simulink model "p2Sim"  (R2019a)
settings: Solver=ode1  StartTime=0.0  StopTime=s.TFinal  FixedStep=s.Tstep  RelTol=1e-3
undefined symbols (not defined in the file): d, kdc, Ki, Kp, mytfpl, s, tau, tau2
settings Model: Creator=vtaware  LastModifiedBy=vtaware

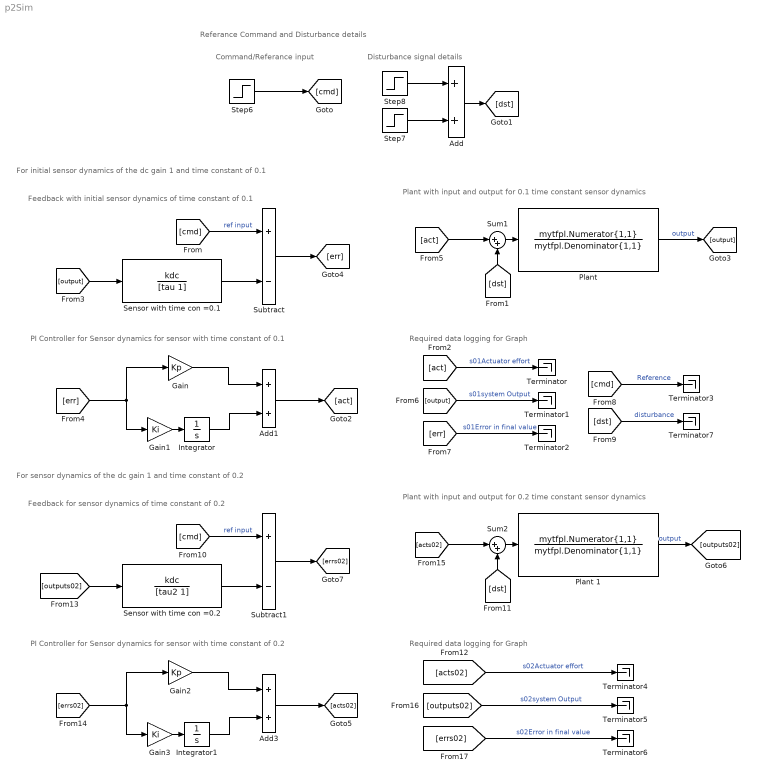
== system p2Sim ==
  note: Referance Command and Disturbance details
  note: Required data logging for Graph
  note: For initial sensor dynamics of the dc gain 1 and time constant of 0.1
  note: Plant with input and output for 0.1 time constant sensor dynamics
  note: Feedback with initial sensor dynamics of time constant of 0.1
  note: PI Controller for Sensor dynamics for sensor with time constant of 0.1
  note: Disturbance signal details
  note: Command/Referance input
  note: Required data logging for Graph
  note: For sensor dynamics of the dc gain 1 and time constant of 0.2
  note: Plant with input and output for 0.2 time constant sensor dynamics
  note: Feedback for sensor dynamics of time constant of 0.2
  note: PI Controller for Sensor dynamics for sensor with time constant of 0.2
  Add : Sum
  Add1 : Sum
  Add3 : Sum
  Gain : Gain  Gain=Kp
  Gain1 : Gain  Gain=Ki
  Gain2 : Gain  Gain=Kp
  Gain3 : Gain  Gain=Ki
  Integrator : Integrator
  Integrator1 : Integrator
  "Plant " : TransferFcn  Numerator=mytfpl.Numerator{1,1}  Denominator=mytfpl.Denominator{1,1}
  Plant 1 : TransferFcn  Numerator=mytfpl.Numerator{1,1}  Denominator=mytfpl.Denominator{1,1}
  Sensor with time con =0.1 : TransferFcn  Numerator=kdc  Denominator=[tau 1]
  Sensor with time con =0.2 : TransferFcn  Numerator=kdc  Denominator=[tau2 1]
  Step6 : Step  Time=s.T0  After=s.A  SampleTime=0
  Step7 : Step  Time=d.T0+d.Tr  After=-d.A  SampleTime=0
  Step8 : Step  Time=d.T0  After=d.A  SampleTime=0
  Subtract : Sum  Inputs=+-
  Subtract1 : Sum  Inputs=+-
  Sum1 : Sum  Inputs=|++
  Sum2 : Sum  Inputs=|++
  Terminator{,1..7} (8 alike) : Terminator
  wires:
  "Plant "/1 -> [output]  "output"
  Sum1/1 -> "Plant "/1
  [err] -> Gain1/1, Gain/1
  Gain1/1 -> Integrator/1
  Step6/1 -> [cmd]
  Step8/1 -> Add/1
  Step7/1 -> Add/2
  Add/1 -> [dst]
  [dst] -> Sum1/2
  Integrator/1 -> Add1/2
  Gain/1 -> Add1/1
  [output] -> Sensor with time con =0.1/1
  [cmd] -> Subtract/1  "ref input"
  Sensor with time con =0.1/1 -> Subtract/2
  Subtract/1 -> [err]
  Add1/1 -> [act]
  [act] -> Sum1/1
  [act] -> Terminator/1  "s01Actuator effort"
  [output] -> Terminator1/1  "s01system Output"
  [err] -> Terminator2/1  "s01Error in final value"
  [cmd] -> Terminator3/1  "Reference"
  [dst] -> Terminator7/1  "disturbance"
  [errs02] -> Terminator6/1  "s02Error in final value"
  [outputs02] -> Terminator5/1  "s02system Output"
  [acts02] -> Terminator4/1  "s02Actuator effort"
  [acts02] -> Sum2/1
  Add3/1 -> [acts02]
  Subtract1/1 -> [errs02]
  Sensor with time con =0.2/1 -> Subtract1/2
  [cmd] -> Subtract1/1  "ref input"
  [outputs02] -> Sensor with time con =0.2/1
  Gain2/1 -> Add3/1
  Integrator1/1 -> Add3/2
  [dst] -> Sum2/2
  Gain3/1 -> Integrator1/1
  [errs02] -> Gain2/1, Gain3/1
  Sum2/1 -> Plant 1/1
  Plant 1/1 -> [outputs02]  "output"
